simulink library "dinr"  (Simulink 8.2)
settings: Solver=ode45  SolverMode=SingleTasking  StartTime=0.0  StopTime=10.0  RelTol=1e-3
undefined symbols (not defined in the file or in its folder): FALSE, KDINR_DisableEstimator_flg, TRUE
libraries: simulink x2
(part 1 of 2)
settings Model: Creator=13192  LastModifiedBy=13192

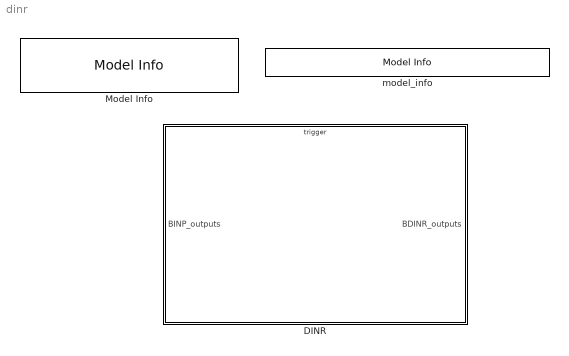
== system dinr ==
  DINR : Subsystem
      settings: RTWSystemCode=Nonreusable function  RTWFcnNameOpts=Use subsystem name  RTWFileNameOpts=Use subsystem name
  Model Info : simulink/Model-Wide Utilities/Model Info  InitialBlockCM=None  BlockCM=None  Frame=on  DisplayStringWithTags=|  HorizontalTextAlignment=Left  LeftAlignmentValue=0.02  SourceBlockDiagram=dinr  TagMaxNumber=20
      | Model Version        : %<ModelVersion>
      | Creator                   : %<Creator>
      | Last Modified by    : %<LastModifiedBy>
  model_info : simulink/Model-Wide Utilities/Model Info  InitialBlockCM=None  BlockCM=None  Frame=on  DisplayStringWithTags=$Id: dinr.mdl 1545 2017-01-16 03:43:29Z bcluan $  HorizontalTextAlignment=Center  LeftAlignmentValue=0.5  SourceBlockDiagram=dinr  TagMaxNumber=20
